simulink model "TwoDOF"  (R2014b)
settings: Solver=ode3  SolverMode=SingleTasking  StartTime=0.0  StopTime=run_time  FixedStep=0.001  RelTol=1e-3
values from neighbouring files (symbols this model uses):
  A = [0 1 0 0 ... (first row only)    [H_inf_ctrl.m]    (also in Hinf_control.m; TwoDOF_mat.m; chassis_passive.m; chassis_skyhook.m)
  B = [0 0 0 0 ... (first row only)    [H_inf_ctrl.m]    (also in Hinf_control.m; TwoDOF_mat.m = [0 0 0; chassis_passive.m; chassis_skyhook.m)
  C = [1 0 0 0 ... (first row only)    [H_inf_ctrl.m]    (also in Hinf_control.m; TwoDOF_mat.m = [1 0 0 0]; chassis_passive.m; chassis_skyhook.m = [0 1 0 0)
  D = [0 0 0 0 ... (first row only)    [H_inf_ctrl.m]    (also in Hinf_control.m; TwoDOF_mat.m = [0 0 0]; chassis_passive.m; chassis_skyhook.m)
  G = ss(Ask,Bsk,Csk,Dsk)    [H_inf_ctrl.m]    (also in TwoDOF_mat.m = minreal(gamma*beta/(alpha*delta-gamma^2)))
  T = 0.08    [TwoDOF_mat.m]
  use_step = 0    [OneDOF_mat.m]    (also in TwoDOF_mat.m = 1; damped_passive_system.m)
settings Model: Creator=signat  LastModifiedBy=eric
settings OptimizationCC: BlockReduction=off  BooleanDataType=off
settings DebuggingCC: SaveWithParameterizedLinksMsg=none  UnderspecifiedInitializationDetection=Classic  MergeDetectMultiDrivingBlocksExec=none  SignalResolutionControl=TryResolveAllWithWarning  SolverPrmCheckMsg=none
settings HardwareCC: TargetUnknown=on

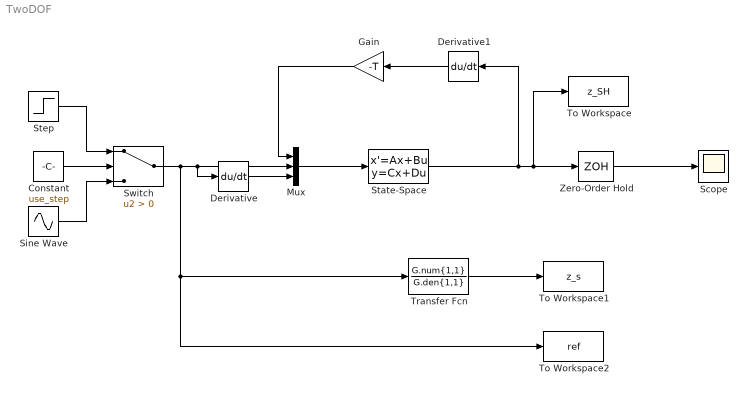
== system TwoDOF ==
  Constant : Constant  Value=use_step
  Derivative : Derivative
  Derivative1 : Derivative
  Gain : Gain  Gain=-T
  Mux : Mux  Inputs=3
  Scope : Scope
  Sine Wave : Sin  Amplitude=0.05  SampleTime=0
  State-Space : StateSpace  A=A  B=B  C=C  D=D  X0=0
  Step : Step  After=0.05  SampleTime=0
  Switch : Switch  Criteria=u2 > Threshold
  To Workspace : ToWorkspace  VariableName=z_SH  SaveFormat=Timeseries  SampleTime=-1
  To Workspace1 : ToWorkspace  VariableName=z_s  SaveFormat=Timeseries  SampleTime=-1
  To Workspace2 : ToWorkspace  VariableName=ref  SaveFormat=Timeseries  SampleTime=-1
  Transfer Fcn : TransferFcn  Numerator=G.num{1,1}  Denominator=G.den{1,1}
  Zero-Order Hold : ZeroOrderHold  SampleTime=0.1
  wires:
  Step/1 -> Switch/1
  Sine Wave/1 -> Switch/3
  Constant/1 -> Switch/2
  State-Space/1 -> To Workspace/1, Zero-Order Hold/1, Derivative1/1
  Derivative/1 -> Mux/3
  Gain/1 -> Mux/1
  Mux/1 -> State-Space/1
  Zero-Order Hold/1 -> Scope/1
  Derivative1/1 -> Gain/1
  Transfer Fcn/1 -> To Workspace1/1
  Switch/1 -> To Workspace2/1, Transfer Fcn/1, Derivative/1, Mux/2
